simulink model "simulation2"  (R2014b)
settings: Solver=ode45  StartTime=0.0  StopTime=10  RelTol=1e-3
values from neighbouring files (symbols this model uses):
  p = d./m    [main2.m]
  q = k./m    [main2.m]
  x_0 = 1    [main2.m]
  x_dot_0 = 0    [main2.m]
settings Model: Creator=rende_000  LastModifiedBy=rende_000

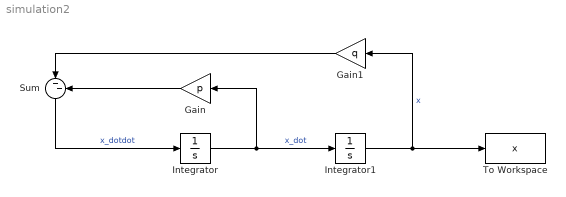
== system simulation2 ==
  Gain : Gain  Gain=p
  Gain1 : Gain  Gain=q
  Integrator : Integrator  InitialCondition=x_dot_0
  Integrator1 : Integrator  InitialCondition=x_0
  Sum : Sum  Inputs=|--
  To Workspace : ToWorkspace  VariableName=x  SaveFormat=Timeseries  SampleTime=-1
  wires:
  Integrator/1 -> Gain/1, Integrator1/1  "x_dot"
  Sum/1 -> Integrator/1  "x_dotdot"
  Integrator1/1 -> To Workspace/1, Gain1/1  "x"
  Gain/1 -> Sum/2
  Gain1/1 -> Sum/1
